simulink model "top_model_rw_desatTest_no_GNC"  (R2018a)
settings: Solver=FixedStepAuto  StartTime=0.0  StopTime=100  FixedStep=.2  RelTol=1e-3  EnableMultiTasking=on
model workspace: external: MATLAB File C:\Users\Stewart\Documents\OAAN\GNC\PAN_ADCS-master\initialization\simulink_workspace_init.m (data not in the file)
undefined symbols (not defined in the file or in its folder): h_init, hdmax, hmax, IAU, Imp_max, Imp_min, init, K_F, Kd, km, Kp, L_F, m_follower, match_tol, muE, ontime_max, ontime_min, q_init, s, Thrust_max, Thrust_min, wbn_init
libraries: aerolibtransform2 x12, aerolibconvert2 x8, sharedtransform x8, hEemethod x8, aerolibgravity2 x6, aerolibutil x6, aerolibcelestial x4, vrlib x4
(part 5 of 5)

== matlab function top_model_rw_desatTest_no_GNC/Attitude Determination and Desired Attitude/Position and Velocity to Desired Attitude in Quat/dcm2quat ==
  data: DCM_be input; q output; tr output; q_prev input; flag output
function [q, tr, flag] = fcn(DCM_be,q_prev)
tr= DCM_be(1,1) + DCM_be(2,2) + DCM_be(3,3);
flag=[0 1];
if (tr > 0)
    S= sqrt(1+tr)*2;
    q4= 0.25 * S;
    q1= (DCM_be(3,2)-DCM_be(2,3))/S;
    q2= (DCM_be(1,3)-DCM_be(3,1))/S;
    q3= (DCM_be(2,1)-DCM_be(1,2))/S;
    q=[q1;q2;q3;q4];
    flag(1)=1;
    
elseif ((DCM_be(1,1)>DCM_be(2,2)) && (DCM_be(1,1)>DCM_be(3,3)))
    S= sqrt(1+DCM_be(1,1)-DCM_be(2,2)-DCM_be(3,3))*2;
    q4= (DCM_be(3,2)-DCM_be(2,3))/S;
    q1= 0.25*S;
    q2= (DCM_be(1,2)+DCM_be(2,1))/S;
    q3= (DCM_be(1,3)+DCM_be(3,1))/S;
    flag(1)=2;
    q=[q1;q2;q3;q4];
elseif (DCM_be(2,2)>DCM_be(3,3))
    S= sqrt(1+DCM_be(2,2)-DCM_be(1,1)-DCM_be(3,3))*2;
    q4= (DCM_be(1,3)-DCM_be(3,1))/S;
    q1= (DCM_be(1,2)+DCM_be(2,1))/S;
    q2= 0.25*S;
    q3= (DCM_be(2,3)+DCM_be(3,2))/S;
    flag(1)=3;
    q=[q1;q2;q3;q4];
else
    S= sqrt(1+DCM_be(3,3)-DCM_be(1,1)-DCM_be(2,2))*2;
    q4= (DCM_be(2,1)-DCM_be(1,2))/S;
    q1= (DCM_be(1,3)+DCM_be(3,1))/S;
    q2= (DCM_be(2,3)+DCM_be(3,2))/S;
    q3= 0.25*S;
    flag(1)=4;
    q=[q1;q2;q3;q4];
end


if  (flag(2)*sign(q(1))*sign(q_prev(1))==-1 && q(1)*q(1)>1e-8) || ...
    (flag(2)*sign(q(2))*sign(q_prev(2))==-1 && q(2)*q(2)>1e-8) || ...
    (flag(2)*sign(q(3))*sign(q_prev(3))==-1 && q(3)*q(3)>1e-8)
    %sign(q_prev(1))==0 || ...
    %sign(q_prev(2))==0 || ...
    %sign(q_prev(3))==0
    
    flag(2)=flag(2)*-1;
end
if flag(2)==-1
    q=-q;
end

== matlab function top_model_rw_desatTest_no_GNC/LDR_Plant/Atmospheric drag ==
  data: velocity input; drag output
function drag = fcn(velocity)
V= norm(velocity);    % 
A= 0.01*0.01;   % 10cm x 10cm
Cd= 0.82;       % for long square cylinder
drag = Cd * A * .5 * 1e-8 * V * -velocity;

== matlab function top_model_rw_desatTest_no_GNC/Controller/Propulsion/MATLAB Function ==
  data: Target input; t_vector1stage output; Best_3_names output; onVec output
%%%Thrust Vector Calculations

%  Input: Vectorized Impulse Requirement (Target) and the thrust vectors on
%  the current nozzle block (Thrust_vectors)

%  Output: 
%   -Thruster On-time vector for the 3 main thrusters
%   -the numbers of the three main thrusters
%   -the on time in terms of thrusters 1,2,3,4

% UNITS of this code is impulse, we take the force vectors of the nozzles
% then scale them accordingly
function [t_vector1stage, Best_3_names, onVec] = get_thruster_onTimes(Target)
    Best_3_names= zeros(3,1);
    % check the input arguments
    [r,c] = size(Target);
    if r~=3 || c~=1
        error('Function argument must be a 3x1 vector')
    end
    % generate the thrust vectors based on the specific nozzle block and
    % the thrust measured per nozzle 
    
    %%% IMPUT THRUST PER NOZZLE %%%
    Thrust_per_nozzle = 5.3E-4; %N
    Thrust_vectors = Generate_Thrust_Vectors(Thrust_per_nozzle); % generates 4x3 matrix 
    
        % determines thrust vectors to be used as a basis in the
        % firing
        angles = zeros(1,4);
        
        % check the angles to each thruster vector
        for i = 1:4 
            angles(i) = acos(dot(Thrust_vectors(:,i),Target)/(norm(Thrust_vectors(:,i))*norm(Target)));
        end

        [~,Indices] = sort(angles);
        
        Best_3_vectors = Thrust_vectors(:,Indices(1:3)); % loads the thruster's vectors
        Best_2_vectors = Thrust_vectors(:,Indices(1:2));
        Best_vector = Thrust_vectors(:,Indices(1));
        
        Best_3_names(1:3) = Indices(1:3); % loads names of the thrusters

        
   % generate on times (2 different methods)
   
   % method 1: 1 stage - 3 thrusters fire in one go, but for different
   % times each, the time vector t_vector1stage gives the thrust for the
   % associated thruster
        
        % x = A\B solves the system of linear equations A*x = B
        t_vector1stage = Best_3_vectors \ Target;
        
        % get the on vector in terms of the nozzles in order
        onVec = zeros(1,4);
        for i = 1:3 % 3 is the number of nozzles given fire orders
            for j = 1:4 % 4 is the number of possible nozzles
                if Best_3_names(i)==j
                   onVec(j) = t_vector1stage(i);
                end
            end

        end

%%%%% METHOD 2 not used as it costs more in terms of opening and closing nozzles and uses the exact same amount of fuel         
%    % method 2: 3 stage
% 
%         bigMat = [ sum(Best_3_vectors,2), sum(Best_2_vectors,2), Best_vector ]; % establishes a vector for three stages with first column as (v1+v2+v3) seoncd (v1+v2), third v1
%         t_vector3stage = bigMat \ Target;


end
%%%Calculate Nozzle Vectors 

function Thrust_vectors = Generate_Thrust_Vectors(Thrust_per_nozzle)

% defined the nozzle block in CAD as Nozzle1, note that each has the
% following sign convention relative to full sat coordinate sytem:
    % Nozzle1:-x+y-z, Nozzle2:+x,-y,-z, Nozzle3:-x,-y,+z, Nozzle4:+x+y+z

% measure the end of the nozzle point in CAD referenced to the Coordinate
% System 2 placed at the hypothetical center of mass of the propulsion
% system in nozzle CAD file, place magnitude of each axis below:

%%% INPUT MEASUREMANTS FROM CADS %%%
magx = 28.3;
magy = 48.73;
magz = 42.402861;
mag_vector = [magx; magy; magz];

% make the vector magnitudes into magnitudes for unit vector
mag_vector_unit = [magx/norm(mag_vector); magy/norm(mag_vector); magz/norm(mag_vector)];
% scale unit vector by the magnitude of the thrust vector
mag_vector_scaled_thrust = mag_vector_unit*Thrust_per_nozzle;
% make the unit vectors for each thruster using sign changes
Nozzle1 = [-mag_vector_scaled_thrust(1);+mag_vector_scaled_thrust(2);-mag_vector_scaled_thrust(3)];
Nozzle2 = [+mag_vector_scaled_thrust(1);-mag_vector_scaled_thrust(2);-mag_vector_scaled_thrust(3)];
Nozzle3 = [-mag_vector_scaled_thrust(1);-mag_vector_scaled_thrust(2);+mag_vector_scaled_thrust(3)];
Nozzle4 = [+mag_vector_scaled_thrust(1);+mag_vector_scaled_thrust(2);+mag_vector_scaled_thrust(3)];

Thrust_vectors = [Nozzle1 Nozzle2 Nozzle3 Nozzle4]; % has the thust vector for each nozzle taking into account thrust per nozzle

end

== matlab function top_model_rw_desatTest_no_GNC/LDR_Plant/DecimalYearIncrement/MATLAB Function ==
  data: DecimalYear output; year input; month input; day input; hour input; minute input; second input
% function DecimalYear
% Calculates decimal year of given date and time. Also considers leap years
% Input: year, month, day, hour, minute, second
% Output: decimal year
function DecimalYear = fcn(year,month,day,hour,minute,second)

for i=1:month-1
    if (month == 1 || month == 3 || month == 5 || month == 7 ...
             || month == 8 || month == 10 || month == 12)
         day= day+31;
    elseif (month == 2)
        if isLeapYear(year)
            day= day+29;
        else
            day= day+28;
        end
    else
        day= day+30;
    end
end
DecimalYear= year ...
            +day/(365+isLeapYear(year))   ...
            +hour/(365+isLeapYear(year))/24 ...
            +minute/(365+isLeapYear(year))/24/60 ...
            +second/(365+isLeapYear(year))/24/3600;
end
        
function logical=isLeapYear(year)
if (rem(year,4)==0)
    if (rem(year,100)==0)
        if (rem(year,400)==0)
            logical=1;
        else
            logical=0;
        end
    else
        logical=1;
    end
else
    logical=0;
end
end

== matlab function top_model_rw_desatTest_no_GNC/GNC/Target Orbit ==
  data: r_t input; x_tgt output; v_t input; r_f input; v_f input; els_t input; els_f input; muE input; K_F input; match_tol input
function x_tgt = x_target(r_t,v_t,r_f,v_f,els_t,els_f,muE,K_F,match_tol)

h_f = cross(r_f,v_f);
E_f = -muE/(2*els_f(1));
ev_f = cross(v_f,h_f)/muE - r_f/norm(r_f);
x_f_current = [h_f;E_f;ev_f];

h_t = cross(r_t,v_t);
E_t = -muE/(2*els_t(1));
ev_t = cross(v_t,h_t)/muE - r_t/norm(r_t);
x_t_current = [h_t;E_t;ev_t];

if(~orb_matched(x_f_current,x_t_current,K_F,match_tol))
    x_tgt = x_t_current;
else
    pos_diff = r_t-r_f;
    vhat = v_f/norm(v_f);
    dr_vbar = dot(vhat,pos_diff)*vhat;
    along_track_sep = norm(dr_vbar);
    follower_ahead = (dot(vhat,pos_diff) < 0);

    if (norm(r_t-r_f) > 500000)
        if (follower_ahead)
            da_tgt = 500;
        else
            da_tgt = -500;
        end
    else
        [da_tgt,~] = decel_step(along_track_sep,follower_ahead);
    end

    a_tgt = els_t(1) + da_tgt;

    [~,~,x_tgt]=phasing_orbit(els_t,a_tgt,muE);
end

== matlab function top_model_rw_desatTest_no_GNC/Attitude Determination and Desired Attitude/Position and Velocity to Desired Attitude in Quat/MATLAB Function ==
  data: DCM_be input; q output
function q = fcn(DCM_be)
tr= DCM_be(1,1) + DCM_be(2,2) + DCM_be(3,3);
th= acos((tr-1)/2);
axis= 0.5/sin(th)*[DCM_be(2,3)-DCM_be(3,2);DCM_be(3,1)-DCM_be(1,3);DCM_be(1,2)-DCM_be(2,1)];
q= [axis*sin(th/2);cos(th/2)];

== matlab function top_model_rw_desatTest_no_GNC/Attitude Determination and Desired Attitude/Attitude Determination/Subsystem/MATLAB Function ==
  data: N_sun input; N_mag input; q_triad output; B_sun input; B_mag input
function q_triad = TRIAD(N_sun, N_mag, B_sun, B_mag)
%Based on time and the location of the spacecraft, the sun and magnetic 
%field vectors in the reference frame N are provided. Based on the sun
%sensor and magnetometer readings, the sun and magnetic field vectors are
%provided in the spacecraft's body frame B. This TRIAD algorithm is very
%straightforward and will not be used on the spacecraft, only for the
%sumulation. B/c the algorithm has the orientation of the same vectors in
%different reference frame, it is able to compute the rotation between
%those reference frames. The algorithm will fail if either of the reference
%vectors or observed vectors are parallel or anti parallel.

% Normalize all vectors (should be normalized already)
N_sun=N_sun/norm(N_sun);
B_sun=B_sun/norm(B_sun);
N_mag=N_mag/norm(N_mag);
B_mag=B_mag/norm(B_mag);

% Ensure all vectors have three components and vectors in the same frame
% are not parallel
if size(N_sun)~=[3 1]
    error('N_sun must be a 3-component column vector')
end

if size(B_sun)~=[3 1]
    error('B_sun must be a 3-component column vector')
end

if size(N_mag)~=[3 1]
    error('N_mag must be a 3-component column vector')
end

if size(B_mag)~=[3 1]
    error('B_mag must be a 3-component column vector')
end

if dot(N_sun,N_mag)==1
    error('Reference frame N vectors can not be parallel')
end

if dot(B_sun,B_mag)==1
    error('Body frame B vectors can not be parallel')
end

% Compute orthonogoal right-handed vectors of reference frame
v1=N_sun;
v2=cross(N_sun,N_mag)/norm(cross(N_sun,N_mag));
v3=cross(v1,v2);

% Compute orthonogoal right-handed vectors of body frame
w1=B_sun;
w2=cross(B_sun,B_mag)/norm(cross(B_sun,B_mag));
w3=cross(w1,w2);

DCM_be=w1(:)*v1(:)'+w3(:)*v3(:)'+w2(:)*v2(:)';
tr= DCM_be(1,1) + DCM_be(2,2) + DCM_be(3,3);
th= acos((tr-1)/2);
axis= 0.5/sin(th)*[DCM_be(2,3)-DCM_be(3,2);DCM_be(3,1)-DCM_be(1,3);DCM_be(1,2)-DCM_be(2,1)];
q_triad= [axis*sin(th/2);cos(th/2)];
%q_triad=dcm2quat(DCM_triad);
% q_temp=DCM_triad;
% q_triad=[q_temp(2) q_temp(3) q_temp(4) q_temp(1)];
end

== stateflow chart top_model_rw_desatTest_no_GNC/Controller/Mode Generator ==
  state Detumble
    entry: mode = 1;
    state High % Child State
      entry: y = 10;
    state Low % Child State
      entry: y = 1;
    (default) -> High % Child State
    Low % Child State -> High % Child State : after(1,sec)
    High % Child State -> Low % Child State : after(1,sec)
  state PowerON_RESET
    entry: mode= 1;
  state LargeAngleSlew
  (default) -> PowerON_RESET : {q_cmd_s= q_cmd;
      | q_body_s= q_body;
      | w_body_s= w_body;}
  PowerON_RESET -> Detumble [order 1] : [w_body >= w_dt]
  PowerON_RESET -> LargeAngleSlew [order 2]
  Detumble -> PowerON_RESET [order 1] : after(5,sec)
  Detumble -> LargeAngleSlew [order 2]
  data: q_body input; q_body_s local; q_cmd_s local; q_cmd input; w_body_s local; w_body input; mode output; w_dt parameter double

== matlab function top_model_rw_desatTest_no_GNC/Attitude Determination and Desired Attitude1/Position and Velocity to Desired Attitude in Quat/MATLAB Function ==
  data: DCM_be input; q output
function q = fcn(DCM_be)
tr= DCM_be(1,1) + DCM_be(2,2) + DCM_be(3,3);
th= acos((tr-1)/2);
axis= 0.5/sin(th)*[DCM_be(2,3)-DCM_be(3,2);DCM_be(3,1)-DCM_be(1,3);DCM_be(1,2)-DCM_be(2,1)];
q= [axis*sin(th/2);cos(th/2)];

== matlab function top_model_rw_desatTest_no_GNC/Attitude Determination and Desired Attitude1/Position and Velocity to Desired Attitude in Quat/dcm2quat ==
  data: DCM_be input; q output; tr output; q_prev input; flag output
function [q, tr, flag] = fcn(DCM_be,q_prev)
tr= DCM_be(1,1) + DCM_be(2,2) + DCM_be(3,3);
flag=[0 1];
if (tr > 0)
    S= sqrt(1+tr)*2;
    q4= 0.25 * S;
    q1= (DCM_be(3,2)-DCM_be(2,3))/S;
    q2= (DCM_be(1,3)-DCM_be(3,1))/S;
    q3= (DCM_be(2,1)-DCM_be(1,2))/S;
    q=[q1;q2;q3;q4];
    flag(1)=1;
    
elseif ((DCM_be(1,1)>DCM_be(2,2)) && (DCM_be(1,1)>DCM_be(3,3)))
    S= sqrt(1+DCM_be(1,1)-DCM_be(2,2)-DCM_be(3,3))*2;
    q4= (DCM_be(3,2)-DCM_be(2,3))/S;
    q1= 0.25*S;
    q2= (DCM_be(1,2)+DCM_be(2,1))/S;
    q3= (DCM_be(1,3)+DCM_be(3,1))/S;
    flag(1)=2;
    q=[q1;q2;q3;q4];
elseif (DCM_be(2,2)>DCM_be(3,3))
    S= sqrt(1+DCM_be(2,2)-DCM_be(1,1)-DCM_be(3,3))*2;
    q4= (DCM_be(1,3)-DCM_be(3,1))/S;
    q1= (DCM_be(1,2)+DCM_be(2,1))/S;
    q2= 0.25*S;
    q3= (DCM_be(2,3)+DCM_be(3,2))/S;
    flag(1)=3;
    q=[q1;q2;q3;q4];
else
    S= sqrt(1+DCM_be(3,3)-DCM_be(1,1)-DCM_be(2,2))*2;
    q4= (DCM_be(2,1)-DCM_be(1,2))/S;
    q1= (DCM_be(1,3)+DCM_be(3,1))/S;
    q2= (DCM_be(2,3)+DCM_be(3,2))/S;
    q3= 0.25*S;
    flag(1)=4;
    q=[q1;q2;q3;q4];
end


if  (flag(2)*sign(q(1))*sign(q_prev(1))==-1 && q(1)*q(1)>1e-8) || ...
    (flag(2)*sign(q(2))*sign(q_prev(2))==-1 && q(2)*q(2)>1e-8) || ...
    (flag(2)*sign(q(3))*sign(q_prev(3))==-1 && q(3)*q(3)>1e-8)
    %sign(q_prev(1))==0 || ...
    %sign(q_prev(2))==0 || ...
    %sign(q_prev(3))==0
    
    flag(2)=flag(2)*-1;
end
if flag(2)==-1
    q=-q;
end

== stateflow chart top_model_rw_desatTest_no_GNC/Controller1/Mode Generator ==
  state Detumble
    entry: mode = 1;
    state High % Child State
      entry: y = 10;
    state Low % Child State
      entry: y = 1;
    (default) -> High % Child State
    Low % Child State -> High % Child State : after(1,sec)
    High % Child State -> Low % Child State : after(1,sec)
  state PowerON_RESET
    entry: mode= 1;
  state LargeAngleSlew
  (default) -> PowerON_RESET : {q_cmd_s= q_cmd;
      | q_body_s= q_body;
      | w_body_s= w_body;}
  PowerON_RESET -> Detumble [order 1] : [w_body >= w_dt]
  PowerON_RESET -> LargeAngleSlew [order 2]
  Detumble -> PowerON_RESET [order 1] : after(5,sec)
  Detumble -> LargeAngleSlew [order 2]
  data: q_body input; q_body_s local; q_cmd_s local; q_cmd input; w_body_s local; w_body input; mode output; w_dt parameter double

== matlab function top_model_rw_desatTest_no_GNC/Controller1/Propulsion/MATLAB Function ==
  data: Target input; t_vector1stage output; Best_3_names output; onVec output
%%%Thrust Vector Calculations

%  Input: Vectorized Impulse Requirement (Target) and the thrust vectors on
%  the current nozzle block (Thrust_vectors)

%  Output: 
%   -Thruster On-time vector for the 3 main thrusters
%   -the numbers of the three main thrusters
%   -the on time in terms of thrusters 1,2,3,4

% UNITS of this code is impulse, we take the force vectors of the nozzles
% then scale them accordingly
function [t_vector1stage, Best_3_names, onVec] = get_thruster_onTimes(Target)
    Best_3_names= zeros(3,1);
    % check the input arguments
    [r,c] = size(Target);
    if r~=3 || c~=1
        error('Function argument must be a 3x1 vector')
    end
    % generate the thrust vectors based on the specific nozzle block and
    % the thrust measured per nozzle 
    
    %%% IMPUT THRUST PER NOZZLE %%%
    Thrust_per_nozzle = 5.3E-4; %N
    Thrust_vectors = Generate_Thrust_Vectors(Thrust_per_nozzle); % generates 4x3 matrix 
    
        % determines thrust vectors to be used as a basis in the
        % firing
        angles = zeros(1,4);
        
        % check the angles to each thruster vector
        for i = 1:4 
            angles(i) = acos(dot(Thrust_vectors(:,i),Target)/(norm(Thrust_vectors(:,i))*norm(Target)));
        end

        [~,Indices] = sort(angles);
        
        Best_3_vectors = Thrust_vectors(:,Indices(1:3)); % loads the thruster's vectors
        Best_2_vectors = Thrust_vectors(:,Indices(1:2));
        Best_vector = Thrust_vectors(:,Indices(1));
        
        Best_3_names(1:3) = Indices(1:3); % loads names of the thrusters

        
   % generate on times (2 different methods)
   
   % method 1: 1 stage - 3 thrusters fire in one go, but for different
   % times each, the time vector t_vector1stage gives the thrust for the
   % associated thruster
        
        % x = A\B solves the system of linear equations A*x = B
        t_vector1stage = Best_3_vectors \ Target;
        
        % get the on vector in terms of the nozzles in order
        onVec = zeros(1,4);
        for i = 1:3 % 3 is the number of nozzles given fire orders
            for j = 1:4 % 4 is the number of possible nozzles
                if Best_3_names(i)==j
                   onVec(j) = t_vector1stage(i);
                end
            end

        end

%%%%% METHOD 2 not used as it costs more in terms of opening and closing nozzles and uses the exact same amount of fuel         
%    % method 2: 3 stage
% 
%         bigMat = [ sum(Best_3_vectors,2), sum(Best_2_vectors,2), Best_vector ]; % establishes a vector for three stages with first column as (v1+v2+v3) seoncd (v1+v2), third v1
%         t_vector3stage = bigMat \ Target;


end
%%%Calculate Nozzle Vectors 

function Thrust_vectors = Generate_Thrust_Vectors(Thrust_per_nozzle)

% defined the nozzle block in CAD as Nozzle1, note that each has the
% following sign convention relative to full sat coordinate sytem:
    % Nozzle1:-x+y-z, Nozzle2:+x,-y,-z, Nozzle3:-x,-y,+z, Nozzle4:+x+y+z

% measure the end of the nozzle point in CAD referenced to the Coordinate
% System 2 placed at the hypothetical center of mass of the propulsion
% system in nozzle CAD file, place magnitude of each axis below:

%%% INPUT MEASUREMANTS FROM CADS %%%
magx = 28.3;
magy = 48.73;
magz = 42.402861;
mag_vector = [magx; magy; magz];

% make the vector magnitudes into magnitudes for unit vector
mag_vector_unit = [magx/norm(mag_vector); magy/norm(mag_vector); magz/norm(mag_vector)];
% scale unit vector by the magnitude of the thrust vector
mag_vector_scaled_thrust = mag_vector_unit*Thrust_per_nozzle;
% make the unit vectors for each thruster using sign changes
Nozzle1 = [-mag_vector_scaled_thrust(1);+mag_vector_scaled_thrust(2);-mag_vector_scaled_thrust(3)];
Nozzle2 = [+mag_vector_scaled_thrust(1);-mag_vector_scaled_thrust(2);-mag_vector_scaled_thrust(3)];
Nozzle3 = [-mag_vector_scaled_thrust(1);-mag_vector_scaled_thrust(2);+mag_vector_scaled_thrust(3)];
Nozzle4 = [+mag_vector_scaled_thrust(1);+mag_vector_scaled_thrust(2);+mag_vector_scaled_thrust(3)];

Thrust_vectors = [Nozzle1 Nozzle2 Nozzle3 Nozzle4]; % has the thust vector for each nozzle taking into account thrust per nozzle

end

== matlab function top_model_rw_desatTest_no_GNC/FWR_Plant/Atmospheric drag ==
  data: velocity input; drag output
function drag = fcn(velocity)
V= norm(velocity);    % 
A= 0.01*0.01;   % 10cm x 10cm
Cd= 0.82;       % for long square cylinder
drag = Cd * A * .5 * 1e-8 * V * -velocity;

== matlab function top_model_rw_desatTest_no_GNC/FWR_Plant/DecimalYearIncrement/MATLAB Function ==
  data: DecimalYear output; year input; month input; day input; hour input; minute input; second input
% function DecimalYear
% Calculates decimal year of given date and time. Also considers leap years
% Input: year, month, day, hour, minute, second
% Output: decimal year
function DecimalYear = fcn(year,month,day,hour,minute,second)

for i=1:month-1
    if (month == 1 || month == 3 || month == 5 || month == 7 ...
             || month == 8 || month == 10 || month == 12)
         day= day+31;
    elseif (month == 2)
        if isLeapYear(year)
            day= day+29;
        else
            day= day+28;
        end
    else
        day= day+30;
    end
end
DecimalYear= year ...
            +day/(365+isLeapYear(year))   ...
            +hour/(365+isLeapYear(year))/24 ...
            +minute/(365+isLeapYear(year))/24/60 ...
            +second/(365+isLeapYear(year))/24/3600;
end
        
function logical=isLeapYear(year)
if (rem(year,4)==0)
    if (rem(year,100)==0)
        if (rem(year,400)==0)
            logical=1;
        else
            logical=0;
        end
    else
        logical=1;
    end
else
    logical=0;
end
end

== matlab function top_model_rw_desatTest_no_GNC/Actuator Model1/Rigid Body with Momentum Actuators and energy dissipation/MATLAB Function ==
  data: hb output; hb_des input; h input; h_min input; temp output; dhdt input
function [hb, temp] = deadband(hb_des,h,h_min,dhdt)

dt = 0.07; % 100 Hz simulation
hb = hb_des; % initialize as desired torque
temp = 0;

% if any element of the desired torque is in the deadband, apply a torque
% that accelerates it to the other side
for k = 1:numel(h)
    if abs(h(k)) < h_min(k)
%         temp = 1;
        if dhdt(k) > 0
            hb(k) = (h_min(k) - h(k))/dt;
        elseif dhdt(k) < 0
            temp = 1;
            hb(k) = (-h_min(k) - h(k))/dt;
        end
    end
end
